simulink model "RUANPANJUE"  (R2016a)
settings: Solver=VariableStepAuto  StartTime=0.0  StopTime=100  RelTol=1e-3
libraries: commcnvcod2 x2, commchan3 x1, commdigbbndpm3 x1, commrandsrc3 x1, commsink2 x1, dspstat3 x1, dspquant2 x1
settings Model: Creator=Administrator  LastModifiedBy=Administrator

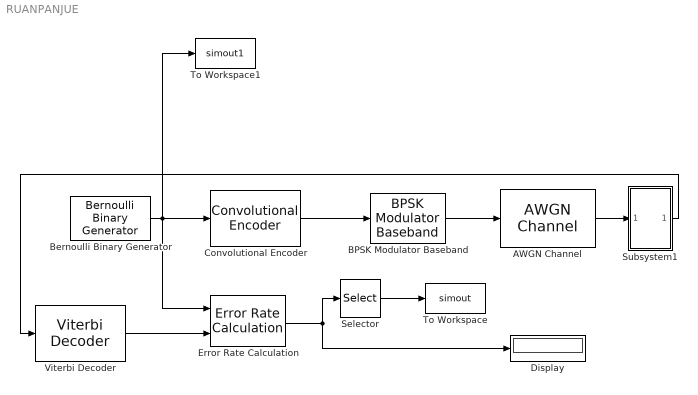
== system RUANPANJUE ==
  AWGN Channel : commchan3/AWGN Channel  InputProcessing=Columns as channels (frame based)  seed=67  noiseMode="Signal to noise ratio  (Eb/No)"  EbNodB=10  EsNodB=10  SNRdB=10  bitsPerSym=1  Ps=1  Tsym=10000  variance=1
  BPSK Modulator Baseband : commdigbbndpm3/BPSK Modulator Baseband  Ph=0  outDtype=double  outWordLen=16  outUDDataType=sfix(16)  outFracLenMode=Best precision  outFracLen=15  outDataTypeStr=double  outLastDataTypeStr=double
  Bernoulli Binary Generator : commrandsrc3/Bernoulli Binary Generator  ProbabilityOfZero=0.4  SeedSource=Auto  Seed=0  SampleTime=100  SamplesPerFrame=10000  OutputDataType=double  SimulateUsing=Interpreted execution
  Convolutional Encoder : commcnvcod2/Convolutional Encoder  trellis=poly2trellis(7, [171 133])  opMode=Continuous  DelayedResetAction=off  hasIniStPort=off  hasFinStPort=off  usePuncVector=off  punctureVector=[1; 1; 0; 1; 0; 1]  reset=Unused parameter value
  Display : Display
  Error Rate Calculation : commsink2/Error Rate Calculation  N=0  st_delay=0  cp_mode=Entire frame  subframe=[]  PMode=Port  WsName=ErrorVec  RsMode2=off  stop=off  numErr=100  maxBits=1e6
  Selector : Selector  IndexMode=Zero-based  InputPortWidth=3  IndexOptions=Index vector (dialog)  Indices=0  OutputSizes=1
  Subsystem1 : Subsystem
  To Workspace : ToWorkspace  VariableName=simout  SaveFormat=Timeseries  SampleTime=-1
  To Workspace1 : ToWorkspace  VariableName=simout1  SaveFormat=Timeseries  SampleTime=-1
  Viterbi Decoder : commcnvcod2/Viterbi Decoder  trellis=poly2trellis(7, [171 133])  isPunctured=off  punctureVector=[1; 1; 0; 1; 0; 1]  erasures=off  dectype=Unquantized  nsdecb=4  runSigValErrCheck=off  tbdepth=34  opmode=Continuous  reset=off  delayedResetAction=off  smWordLength=16  outDataType=Inherit via internal rule
  wires:
  Bernoulli Binary Generator/1 -> To Workspace1/1, Error Rate Calculation/1, Convolutional Encoder/1
  Convolutional Encoder/1 -> BPSK Modulator Baseband/1
  BPSK Modulator Baseband/1 -> AWGN Channel/1
  Viterbi Decoder/1 -> Error Rate Calculation/2
  AWGN Channel/1 -> Subsystem1/1(In1)
  Subsystem1/1(Out1) -> Viterbi Decoder/1
  Error Rate Calculation/1 -> Display/1, Selector/1
  Selector/1 -> To Workspace/1

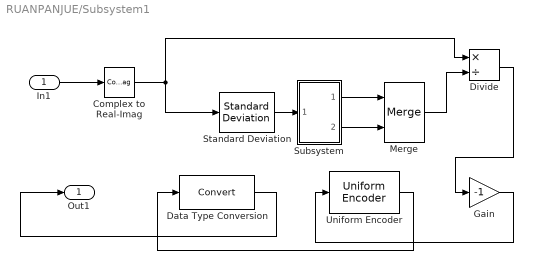
== system RUANPANJUE/Subsystem1 ==
  In1 : Inport
  Complex to Real-Imag : ComplexToRealImag  Output=Real
  Data Type Conversion : DataTypeConversion
  Divide : Product  Inputs=*/
  Gain : Gain  Gain=-1
  Merge : Merge
  Standard Deviation : dspstat3/Standard Deviation  run=off  reset_popup=None  InputProcessing=Columns as channels (frame based)  directionMode=Each column  dimension=1  roiEnable=off  roiType=Rectangles  roiPortion=Entire ROI  roiOutput=Individual statistics for each ROI  roiFlag=off
  Subsystem : Subsystem
  Uniform Encoder : dspquant2/Uniform Encoder  peak=2  bits=3  otype=Unsigned integer
  Out1 : Outport
  wires:
  Complex to Real-Imag/1 -> Divide/1, Standard Deviation/1
  Subsystem/1(Out1) -> Merge/1
  Gain/1 -> Uniform Encoder/1
  Uniform Encoder/1 -> Data Type Conversion/1
  In1/1 -> Complex to Real-Imag/1
  Data Type Conversion/1 -> Out1/1
  Divide/1 -> Gain/1
  Standard Deviation/1 -> Subsystem/1(In1)
  Merge/1 -> Divide/2
  Subsystem/2(Out2) -> Merge/2

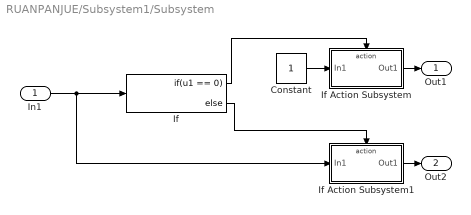
== system RUANPANJUE/Subsystem1/Subsystem ==
  In1 : Inport
  Constant : Constant
  If : If  IfExpression=u1 == 0
  If Action Subsystem : Subsystem  TreatAsAtomicUnit=on
  If Action Subsystem1 : Subsystem  TreatAsAtomicUnit=on
  Out1 : Outport
  Out2 : Outport  Port=2
  wires:
  Constant/1 -> If Action Subsystem/1(In1)
  In1/1 -> If Action Subsystem1/1(In1), If/1
  If/1 -> If Action Subsystem/Action
  If Action Subsystem/1(Out1) -> Out1/1
  If Action Subsystem1/1(Out1) -> Out2/1
  If/2 -> If Action Subsystem1/Action

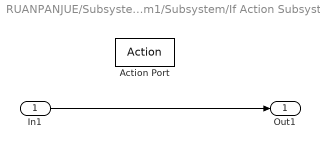
== system RUANPANJUE/Subsystem1/Subsystem/If Action Subsystem ==
  In1 : Inport
  Action Port : ActionPort  ActionType=then
  Out1 : Outport
  wires:
  In1/1 -> Out1/1

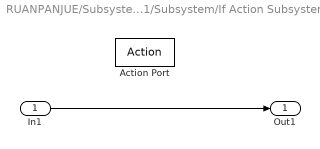
== system RUANPANJUE/Subsystem1/Subsystem/If Action Subsystem1 ==
  In1 : Inport
  Action Port : ActionPort  ActionType=else
  Out1 : Outport
  wires:
  In1/1 -> Out1/1
